simulink model "cicexample1_sim"  (R2022a)
settings: Solver=FixedStepDiscrete  StartTime=0.0  StopTime=Tstop  RelTol=1e-3  EnableMultiTasking=on
values from neighbouring files (symbols this model uses):
  dec = 256    [CIC_scriptexample1.m]    (also in Sigmadelta_1bit_CIC.m = 128)
  Ts = 1/Fs    (= 1.6e-05)    [CIC_scriptexample1.m]
undefined symbols (not defined in the file or in its folder): order
settings Model: Creator=ceballos  LastModifiedBy=eduyilmet001
settings SolverCC: AlgebraicLoopSolver=TrustRegion
settings DataIOCC: LimitDataPoints=on  SaveFormat=Array  SignalLoggingSaveFormat=ModelDataLogs  ReturnWorkspaceOutputs=off
settings OptimizationCC: BooleanDataType=off  ExpressionDepthLimit=2147483647  LifeSpan=inf
settings DebuggingCC: SaveWithParameterizedLinksMsg=none  UnderspecifiedInitializationDetection=Classic  MergeDetectMultiDrivingBlocksExec=none  SignalResolutionControl=TryResolveAllWithWarning  MultiTaskDSMMsg=warning  MultiTaskCondExecSysMsg=none  FcnCallInpInsideContextMsg=warning  UnconnectedInputMsg=warning  UnconnectedOutputMsg=warning  UnconnectedLineMsg=warning  StateNameClashWarn=warning  SFUnexpectedBacktrackingDiag=warning  SFNoUnconditionalDefaultTransitionDiag=warning  SFExecutionAtInitializationDiag=none  SFMachineParentedDataDiag=warning  ArithmeticOperatorsInVariantConditions=warning
settings HardwareCC: ProdBitPerPointer=32  ProdBitPerSizeT=32  ProdBitPerPtrDiffT=32  ProdLargestAtomicFloat=None  ProdIntDivRoundTo=Undefined  ProdEndianess=Unspecified  ProdWordSize=32  ProdHWDeviceType=32-bit Generic  TargetBitPerPointer=64  TargetBitPerSizeT=64  TargetBitPerPtrDiffT=64  TargetLongLongMode=on  TargetIntDivRoundTo=Zero  TargetEndianess=LittleEndian  TargetWordSize=64  TargetHWDeviceType=MATLAB Host  ProdEqTarget=off
settings ModelReferenceCC: PropagateSignalLabelsOutOfModel=off
settings SFSimCC: SimUseLocalCustomCode=off  CustomCodeUndefinedFunction=UseInterfaceOnly
settings RTWCC: RTWUseLocalCustomCode=off  DLArmComputeVersion=19.05
settings CodeAppCC: StateflowObjectComments=on
settings GRTTargetCC: TargetLangStandard=C89/C90 (ANSI)  CombineOutputUpdateFcns=off  GRTInterface=on
settings ConfigComp: CovMetricSettings=dw  CovSaveCumulativeToWorkspaceVar=on  CovSaveSingleToWorkspaceVar=on  CovExternalEMLEnable=off  CovSFcnEnable=off

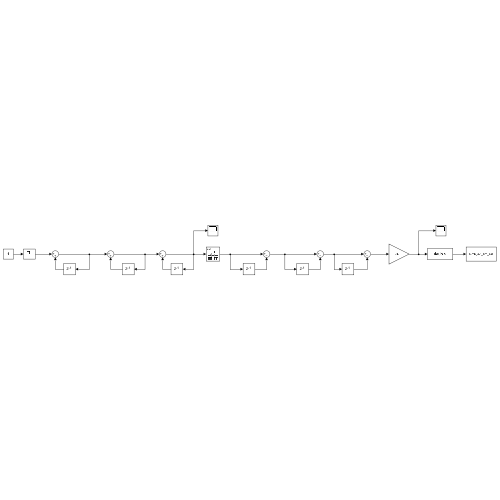
[thumbnail: Simulink's stored preview of the top-level diagram]
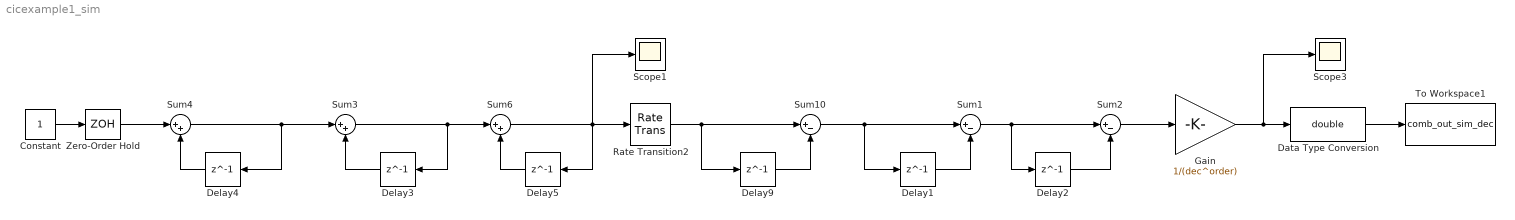
== system cicexample1_sim ==
  Constant : Constant  OutDataTypeStr=fixdt(1,5,0)  SampleTime=Ts
  Data Type Conversion : DataTypeConversion  OutDataTypeStr=double  SaturateOnIntegerOverflow=off  RndMeth=Floor
  Delay{1..5,9} (6 alike) : Delay  DelayLength=1  InitialCondition=0
  Gain : Gain  Gain=1/(dec^order)
  Rate Transition2 : RateTransition  OutPortSampleTimeOpt=Multiple of input port sample time  OutPortSampleTimeMultiple=dec
  Scope1 : Scope
  Scope3 : Scope
  Sum1 : Sum  Inputs=|+-  AccumDataTypeStr=fixdt(1,26,0)  OutDataTypeStr=Inherit: Same as accumulator
  Sum10 : Sum  Inputs=|+-  AccumDataTypeStr=fixdt(1,26,0)  OutDataTypeStr=Inherit: Same as accumulator
  Sum2 : Sum  Inputs=|+-  AccumDataTypeStr=fixdt(1,26,0)  OutDataTypeStr=Inherit: Same as accumulator
  Sum3 : Sum  Inputs=|++  AccumDataTypeStr=fixdt(1,26,0)  OutDataTypeStr=Inherit: Same as accumulator
  Sum4 : Sum  Inputs=|++  AccumDataTypeStr=fixdt(1,26,0)  OutDataTypeStr=Inherit: Same as accumulator
  Sum6 : Sum  Inputs=|++  AccumDataTypeStr=fixdt(1,26,0)  OutDataTypeStr=Inherit: Same as accumulator
  To Workspace1 : ToWorkspace  VariableName=comb_out_sim_dec  SampleTime=-1
  Zero-Order Hold : ZeroOrderHold  SampleTime=Ts
  wires:
  Rate Transition2/1 -> Sum10/1, Delay9/1
  Delay9/1 -> Sum10/2
  Delay5/1 -> Sum6/2
  Data Type Conversion/1 -> To Workspace1/1
  Gain/1 -> Data Type Conversion/1, Scope3/1
  Constant/1 -> Zero-Order Hold/1
  Sum6/1 -> Rate Transition2/1, Scope1/1, Delay5/1
  Sum10/1 -> Delay1/1, Sum1/1
  Delay1/1 -> Sum1/2
  Sum1/1 -> Delay2/1, Sum2/1
  Delay2/1 -> Sum2/2
  Sum2/1 -> Gain/1
  Sum3/1 -> Delay3/1, Sum6/1
  Zero-Order Hold/1 -> Sum4/1
  Sum4/1 -> Delay4/1, Sum3/1
  Delay4/1 -> Sum4/2
  Delay3/1 -> Sum3/2
